simulink subsystem "llh2xyz"  (R2021a)
settings: Solver=VariableStepAuto  StartTime=0.0  StopTime=10.0  RelTol=1e-3
settings Model: Creator=zurnmar  LastModifiedBy=zurnmar

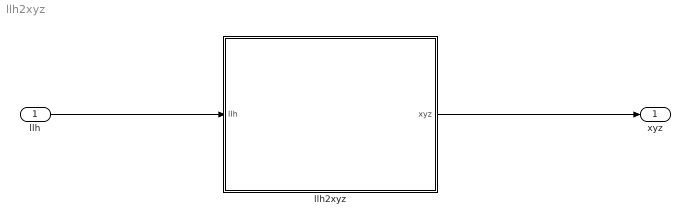
== system llh2xyz ==
  llh : Inport  PortDimensions=[3,1]
  llh2xyz : Subsystem  Description=|  TreatAsAtomicUnit=on  RTWFcnName=llh2xyz
      | <strong> FUNCTION </strong>
      |    This module converts the geodetic WGS84 coordinates to ECEF (Described in Sec.2.5.1)
      |    
      |    @param[in] llh => WGS84 coordinates in Latitude[rad], Longitude[rad], height[m]
      |    
      |    @param[out] xyz => ECEF coordinates in x[m], y[m], z[m]
      |    
      |    <strong>  Constant </strong>
      |    <table>
      |    <tr><th> Label                      <th>Value <th>Description
      |    <tr><td> a    <td>6378137.0			<td>Semi-
      |    <tr><td> b    <td>6356752.3142		<td>Se
      |    <tr><td> e2   <td>0.006694380004261	<td>Eccentricity (e) of the ellipsoid squared (e2=1-b^2/a^2)
      | 
      | @file
      settings: RTWFcnNameOpts=User specified  RTWFileNameOpts=Use function name
  "xyz " : Outport
  wires:
  llh/1 -> llh2xyz/1(llh)
  llh2xyz/1(xyz) -> "xyz "/1

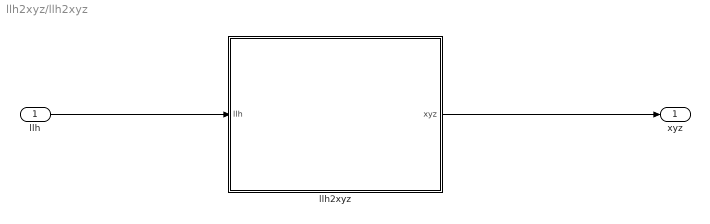
== system llh2xyz/llh2xyz ==
  llh : Inport
  llh2xyz : MATLAB Function  RTWFcnName=llh2xyz
      settings: RTWFileNameOpts=Use function name
  xyz : Outport
  wires:
  llh2xyz/1(xyz) -> xyz/1
  llh/1 -> llh2xyz/1(llh)

== matlab function llh2xyz/llh2xyz ==
  data: llh input; xyz output
function xyz  = llh2xyz(llh)
% WGS84 parameters
% a: semi-major axis
xyz=zeros(3,1);
a = 6378137;
% f: flattening 
f = 1/298.257223563;
% b: semi-minor axis [b=a(1-f)]
% b = 6356752.314245179;

e2 = f*(2-f);
v = a ./ sqrt(1-e2*sin(llh(1,1)).^2);

xyz(1,1) = (v+llh(3,1)) .* cos(llh(1,1)) .* cos(llh(2,1));
xyz(2,1) = (v+llh(3,1)) .* cos(llh(1,1)) .* sin(llh(2,1));
xyz(3,1) = (v*(1-e2)+llh(3,1)) .* sin(llh(1,1));
end
